simulink model "mixer"  (Simulink 7.5)
settings: Solver=ode45  StartTime=0.0  StopTime=10.0  RelTol=1e-6
settings Model: Creator=Ben  LastModifiedBy=Ben

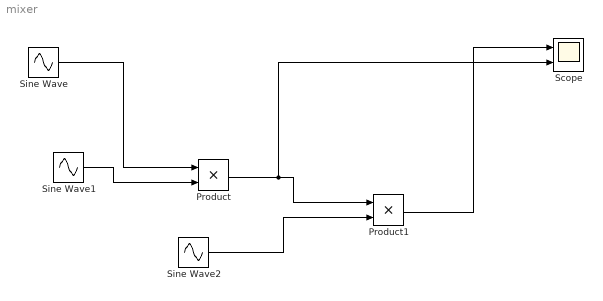
== system mixer ==
  Product : Product  OutDataType=fixdt(1, 16)  OutScaling=2^0  RndMeth=Zero
  Product1 : Product  OutDataType=fixdt(1, 16)  OutScaling=2^0  RndMeth=Zero
  Scope : Scope  NumInputPorts=2
      settings: YMin=-5~-5  YMax=5~5
  Sine Wave : Sin  Amplitude=1  Bias=0  Frequency=2*pi  Phase=0  Samples=10  SampleTime=.001  Offset=0
  Sine Wave1 : Sin  Amplitude=1  Bias=0  Frequency=1  Phase=0  Samples=10  SampleTime=.001  Offset=0
  Sine Wave2 : Sin  Amplitude=1  Bias=0  Frequency=1  Phase=pi/2  Samples=10  SampleTime=.001  Offset=0
  wires:
  Sine Wave/1 -> Product/1
  Sine Wave1/1 -> Product/2
  Product/1 -> Product1/1, Scope/2
  Product1/1 -> Scope/1
  Sine Wave2/1 -> Product1/2
